simulink model "lr5mod"  (R2024a)
settings: Solver=VariableStepAuto  StartTime=0.0  StopTime=0.1  MaxStep=1e-5  RelTol=1e-5
undefined symbols (not defined in the file): DC, f_nes, Nagr, U_mod, UB, w_preobr
libraries: spsFourierLib x4, spsCurrentMeasurementLib x2, spsGroundLib x2, spsDCVoltageSourceLib x1, spsMultimeterLib x1, spsRMSLib x1, spsSeriesRLCBranchLib x1, simulink x1, spsUniversalBridgeLib x1, spsVoltageMeasurementLib x1, sps_lib x1
settings Model: Creator=79532  LastModifiedBy=79532

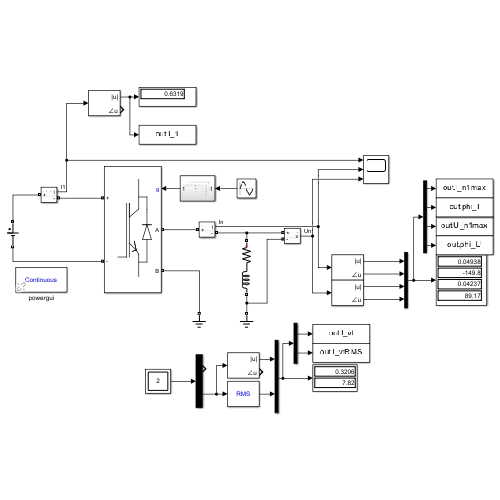
[thumbnail: Simulink's stored preview of the top-level diagram]
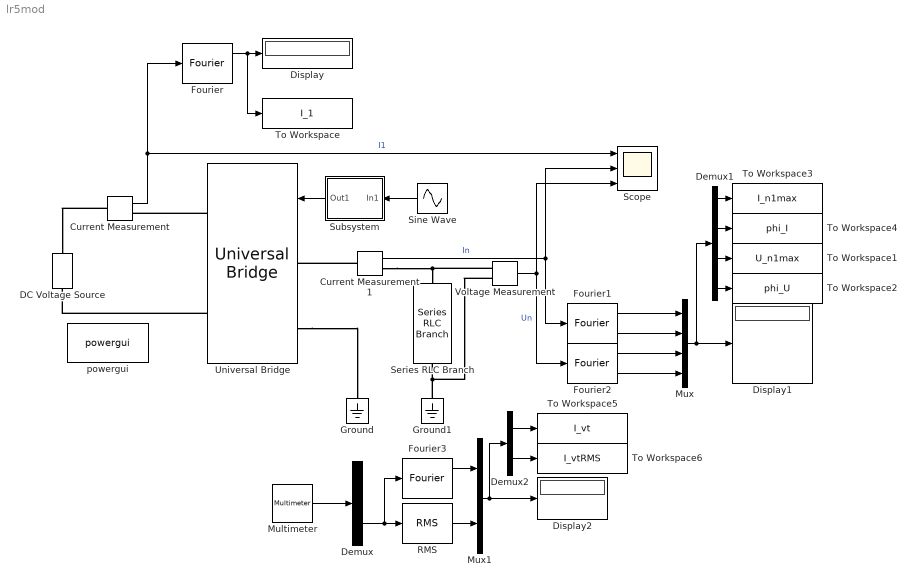
== system lr5mod ==
  Current Measurement : spsCurrentMeasurementLib/Current Measurement  PhasorSimulation=off  OutputType=Complex  PSBequivalent=0
  Current Measurement1 : spsCurrentMeasurementLib/Current Measurement  PhasorSimulation=off  OutputType=Complex  PSBequivalent=0
  DC Voltage Source : spsDCVoltageSourceLib/DC Voltage Source  Amplitude=DC.Voltage  Measurements=None
  Demux : Demux  Outputs=2
  Demux1 : Demux
  Demux2 : Demux  Outputs=2
  Display : Display
  Display1 : Display
  Display2 : Display
  Fourier : spsFourierLib/Fourier  Freq=f_preobr  n=0  InInit=[0, 0]  Ts=0
  Fourier1 : spsFourierLib/Fourier  Freq=f_preobr  n=1  InInit=[0, 0]  Ts=0
  Fourier2 : spsFourierLib/Fourier  Freq=f_preobr  n=1  InInit=[0, 0]  Ts=0
  Fourier3 : spsFourierLib/Fourier  Freq=f_preobr  n=0  InInit=[0, 0]  Ts=0
  Ground : spsGroundLib/Ground  LConnTagsString=a
  Ground1 : spsGroundLib/Ground  LConnTagsString=a
  Multimeter : spsMultimeterLib/Multimeter  L=10  sel=[1 7]  yselected={}  Gain=[1 1]  OutputType=Complex  PlotAtSimulationStop=on  PhasorSimulation=off
  Mux : Mux
  Mux1 : Mux  Inputs=2
  RMS : spsRMSLib/RMS  TrueRMS=on  Freq=f_preobr  RMSInit=0  Ts=0
  Scope : Scope  NumInputPorts=3
  Series RLC Branch : spsSeriesRLCBranchLib/Series RLC Branch  LConnTagsString=__new0  RConnTagsString=__new0  BranchType=RL  Resistance=Nagr.Res  Inductance=Nagr.Ind  SetiL0=off  InitialCurrent=0  Capacitance=1e-6  Setx0=off  InitialVoltage=0  Measurements=None
  Sine Wave : Sin  Amplitude=U_mod  Frequency=w_preobr  SampleTime=0
  Subsystem : Subsystem
  To Workspace : ToWorkspace  VariableName=I_1  SaveFormat=Timeseries  SampleTime=-1
  To Workspace1 : ToWorkspace  VariableName=U_n1max  SaveFormat=Timeseries  SampleTime=-1
  To Workspace2 : ToWorkspace  VariableName=phi_U  SaveFormat=Timeseries  SampleTime=-1
  To Workspace3 : ToWorkspace  VariableName=I_n1max  SaveFormat=Timeseries  SampleTime=-1
  To Workspace4 : ToWorkspace  VariableName=phi_I  SaveFormat=Timeseries  SampleTime=-1
  To Workspace5 : ToWorkspace  VariableName=I_vt  SaveFormat=Timeseries  SampleTime=-1
  To Workspace6 : ToWorkspace  VariableName=I_vtRMS  SaveFormat=Timeseries  SampleTime=-1
  Universal Bridge : spsUniversalBridgeLib/Universal Bridge  Arms=2  SnubberResistance=1e5  SnubberCapacitance=inf  Device=IGBT / Diodes  Ron=UB.R_on  Lon=0  ForwardVoltages="[  UB.V_f  UB.V_fd  ]"  ForwardVoltage=0  GTOparameters=[ 10e-6 , 20e-6 ]  IGBTparameters=[ 1e-6 , 2e-6 ]  Measurements=All voltages and currents  Measurements_2=None  converterType=Rectifier
  Voltage Measurement : spsVoltageMeasurementLib/Voltage Measurement  PhasorSimulation=off  OutputType=Complex  PSBequivalent=0
  powergui : sps_lib/powergui  Priority=1  SimulationMode=Continuous  SampleTime=50e-6  frequency=60  Iterations=50  frequencyindice=0  Pbase=100e6  ErrMax=1e-4  UnitsV=kV  UnitsW=MW  buscounter=0  FunctionMessages=off  echomessages=off  EnableUseOfTLC=off  CurrentSourceSwitches=off  DisableSnubberDevices=off  DisableRonSwitches=off  DisableVfSwitches=off  DisplayEquations=off  AutomaticDiscreteSolvers=off  SolverType=Tustin/Backward Euler (TBE)  Interpol=off  ExternalGateDelay=off  methode=off  Ts=100  x0status=blocks  SPID=on  SwTol=0  HookPort=off  NonlinearTolerance=1e-4  nMaxIteration=100  ContinueOnMaxIteration=off  RestoreLinks=warning  ResistiveCurrentMeasurement=off  Frange=[0:2:500]  Ylog=off  Xlog=on  ShowGrid=off  save=off  variable=ZData  structure=0  ZoomFFT=off  StartTime=0.0  cycles=1  DisplayStyle=1  fundamental=60  FreqAxis=off  MaxFrequency=1000  frequencyindicesteady=1  RmsSteady=1  display=off
  wires:
  Sine Wave/1 -> Subsystem/1(In1)
  Subsystem/1(Out1) -> Universal Bridge/1
  Current Measurement/1 -> Scope/1, Fourier/1  "I1"
  Fourier/1 -> To Workspace/1, Display/1
  Current Measurement1/1 -> Fourier1/1, Scope/2  "In"
  Voltage Measurement/1 -> Fourier2/1, Scope/3  "Un"
  Fourier1/1 -> Mux/1
  Fourier1/2 -> Mux/2
  Fourier2/1 -> Mux/3
  Fourier2/2 -> Mux/4
  Mux/1 -> Demux1/1, Display1/1
  Multimeter/1 -> Demux/1
  Demux/2 -> Fourier3/1, RMS/1
  RMS/1 -> Mux1/2
  Fourier3/1 -> Mux1/1
  Mux1/1 -> Demux2/1, Display2/1
  Demux1/4 -> To Workspace2/1
  Demux1/3 -> To Workspace1/1
  Demux1/2 -> To Workspace4/1
  Demux1/1 -> To Workspace3/1
  Demux2/1 -> To Workspace5/1
  Demux2/2 -> To Workspace6/1
  connections:
  Current Measurement/LConn1 -- DC Voltage Source/RConn1
  Universal Bridge/RConn1 -- Current Measurement/RConn1
  Universal Bridge/RConn2 -- DC Voltage Source/LConn1
  Universal Bridge/LConn2 -- Ground/LConn1
  Ground1/LConn1 -- Voltage Measurement/LConn2 -- Series RLC Branch/RConn1
  Current Measurement1/LConn1 -- Universal Bridge/LConn1
  Current Measurement1/RConn1 -- Voltage Measurement/LConn1 -- Series RLC Branch/LConn1

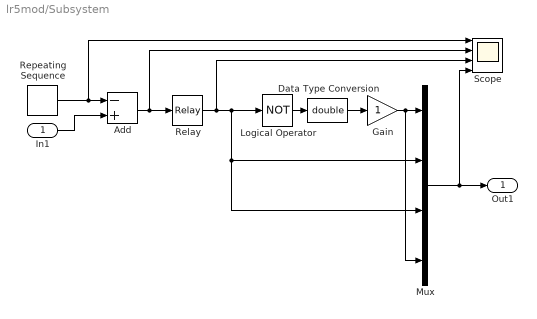
== system lr5mod/Subsystem ==
  In1 : Inport
  Add : Sum  Inputs=-+
  Data Type Conversion : DataTypeConversion  OutDataTypeStr=double  SaturateOnIntegerOverflow=off  RndMeth=Floor
  Gain : Gain
  Logical Operator : Logic  Operator=NOT  AllPortsSameDT=off  OutDataTypeStr=boolean
  Mux : Mux
  Relay : Relay
  Repeating Sequence : simulink/Sources/Repeating Sequence  rep_seq_t=[0 1/2/f_nes 1/f_nes]  rep_seq_y=[-2 2 -2]
  Scope : Scope  NumInputPorts=4
  Out1 : Outport
  wires:
  Relay/1 -> Logical Operator/1, Mux/3, Mux/2, Scope/3
  In1/1 -> Add/2
  Add/1 -> Scope/2, Relay/1
  Repeating Sequence/1 -> Scope/1, Add/1
  Gain/1 -> Mux/4, Mux/1
  Mux/1 -> Out1/1, Scope/4
  Logical Operator/1 -> Data Type Conversion/1
  Data Type Conversion/1 -> Gain/1
